simulink model "sampleModel1568"  (R2023a)
settings: Solver=VariableStepAuto  StartTime=0.0  StopTime=10.0  RelTol=1e-3
libraries: hdlsllib x6, simulink x2
settings Model: Creator=user1  LastModifiedBy=user1

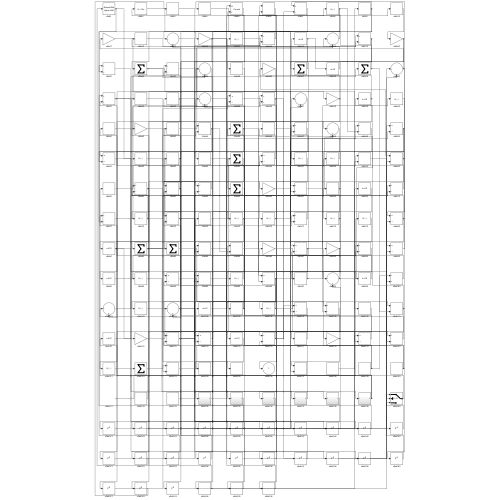
[thumbnail: Simulink's stored preview of the top-level diagram]
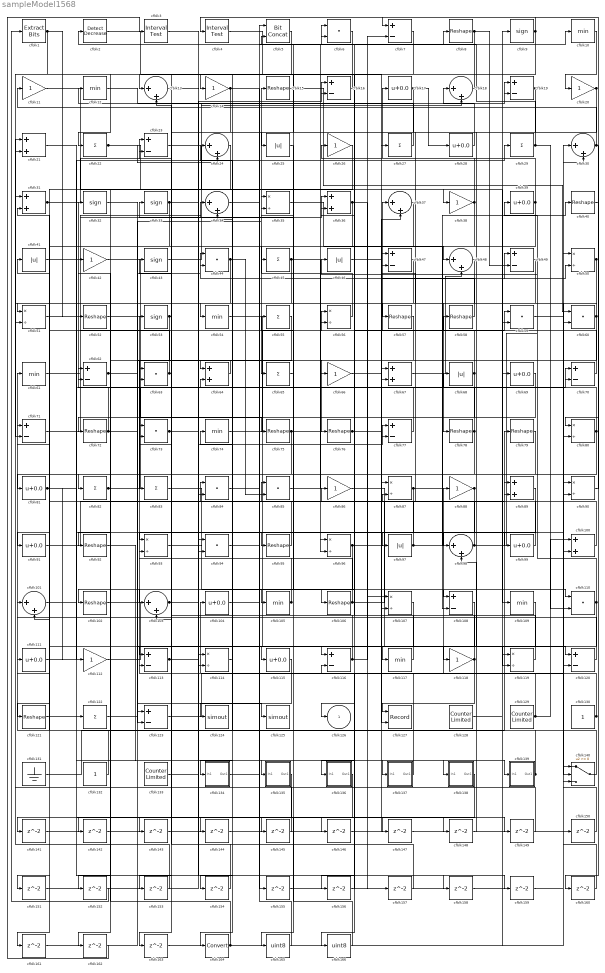
== system sampleModel1568 ==
  cfblk1 : simulink/Logic and Bit Operations/Extract Bits  bitsToExtract=Upper half  numBits=8  bitIdxRange=[0 7]  outScalingMode=Preserve fixed-point scaling
      settings: LibrarySourceBlock=|
      | hdlsllib/Logic and Bit
      | Operations/Extract Bits
  cfblk{10,12,54,61,74,105,109,117} (8 alike) : MinMax
  cfblk{21,31,36,64,67,89,100} (7 alike) : Sum
  cfblk{13,18,24,30,34,37,48,98,101,103} (10 alike) : Sum  Inputs=|++
  cfblk{8,15,40,52,57..58,72,75..76,78..79,92,95,102,106,121} (16 alike) : Reshape
  cfblk{17,28,39,69,81,91,99,104,111,115} (10 alike) : Bias  Bias=0.0  SaturateOnIntegerOverflow=off
  cfblk{35,50..51,56,80,87,90,93,96,107,114,119} (12 alike) : Product  Inputs=*/  RndMeth=Zero  SaturateOnIntegerOverflow=on
  cfblk{7,16,19,23,47,49,62,70..71,77,108,113,116,120,123} (15 alike) : Sum  Inputs=+-
  cfblk{11,14,20,26,38,42,66,86,88,112,118} (11 alike) : Gain
  cfblk{6,44,59..60,63,73,84..85,94,110} (10 alike) : DotProduct  OutDataTypeStr=Inherit: Inherit via internal rule
  cfblk{22,27,29,45,55,65,82..83,122} (9 alike) : Sum  Inputs=+
  cfblk124 : ToWorkspace  VariableName=simout  SaveFormat=Timeseries  SampleTime=-1
  cfblk125 : ToWorkspace  VariableName=simout  SaveFormat=Timeseries  SampleTime=-1
  cfblk127 : Record  FileSettingsInternal="{\"entries\":[{\"content\":{\"excelSettings\":{\"content\":{},\"type\":\"Streamout.ExcelSettings\"}},\"type\":\"Streamout.FileSettingStorage\",\"uuid\":\"\"}],\"packageUris\":[\"http:\\/\\/schema.mathworks.com\\/mf0\\/streamout_blocks\\/R2020a\"],\"version\":\"1.0\"}"  Layout=[1 1]  SignalsInternal="{\"entries\":[{\"content\":{},\"type\":\"RecordBlkView.InputSignals\",\"uuid\":\"\"}],\"packageUris\":[\"http:\\/\\/schema.mathworks.com\\/mf0\\/streamout_blocks\\/R2020a\"],\"version\":\"1.0\"}"  VisualizationBindings="{\"xyplotplugin\":{\"info\":[{\"series\":[{\"bindingParametersList\":[{\"parameter\":\"X-Axis\",\"signalID\":1822,\"signalName\":\"cfblk118\"},{\"parameter\":\"Y-Axis\",\"signalID\":1826,\"signalName\":\"cfblk49\"}],\"seriesID\":63146}],\"subplotID\":1}]}}"  CompatibilityTag=XY  st=-1
  cfblk128 : hdlsllib/Sources/Counter Limited  uplimit=7  tsamp=-1
  cfblk129 : hdlsllib/Sources/Counter Limited  uplimit=7  tsamp=-1
  cfblk130 : Constant  SampleTime=-1
  cfblk131 : Ground
  cfblk132 : Constant  SampleTime=-1
  cfblk133 : hdlsllib/Sources/Counter Limited  uplimit=7  tsamp=-1
  cfblk134 : Subsystem
      settings: LibrarySourceBlock=|
      | hdlsllib/Ports &
      | Subsystems/Subsystem
  cfblk135 : Subsystem
      settings: LibrarySourceBlock=|
      | hdlsllib/Ports &
      | Subsystems/Subsystem
  cfblk136 : Subsystem
      settings: LibrarySourceBlock=|
      | hdlsllib/Ports &
      | Subsystems/Subsystem
  cfblk137 : Subsystem
      settings: LibrarySourceBlock=|
      | hdlsllib/Ports &
      | Subsystems/Subsystem
  cfblk138 : Subsystem
      settings: LibrarySourceBlock=|
      | hdlsllib/Ports &
      | Subsystems/Subsystem
  cfblk139 : Subsystem
      settings: LibrarySourceBlock=|
      | hdlsllib/Ports &
      | Subsystems/Subsystem
  cfblk140 : Switch  SaturateOnIntegerOverflow=off  InputSameDT=off
  cfblk{141..163} (23 alike) : Delay  SampleTime=1
  cfblk164 : DataTypeConversion  SaturateOnIntegerOverflow=off  RndMeth=Floor
  cfblk165 : DataTypeConversion  OutDataTypeStr=uint8  SaturateOnIntegerOverflow=off  RndMeth=Floor
  cfblk166 : DataTypeConversion  OutDataTypeStr=uint8  SaturateOnIntegerOverflow=off  RndMeth=Floor
  cfblk2 : simulink/Logic and Bit Operations/Detect Decrease  vinit=0.0  OutDataTypeStr=boolean
      settings: LibrarySourceBlock=|
      | hdlsllib/Logic and Bit
      | Operations/Detect
      | Decrease
  cfblk{25,41,46,68,97} (5 alike) : Abs  SaturateOnIntegerOverflow=off
  cfblk3 : hdlsllib/Logic and Bit Operations/Interval Test  IntervalClosedRight=on  uplimit=0.5  IntervalClosedLeft=on  lowlimit=-0.5  OutDataTypeStr=boolean
  cfblk{9,32..33,43,53} (5 alike) : Signum
  cfblk4 : hdlsllib/Logic and Bit Operations/Interval Test  IntervalClosedRight=on  uplimit=0.5  IntervalClosedLeft=on  lowlimit=-0.5  OutDataTypeStr=boolean
  cfblk5 : hdlsllib/Logic and Bit Operations/Bit Concat  numInputs=2
  cfblk126 : Outport  VectorParamsAs1DForOutWhenUnconnected=off
  wires:
  cfblk54/1 -> cfblk120/1
  cfblk31/1 -> cfblk23/1, cfblk97/1
  cfblk77/1 -> cfblk33/1
  cfblk129/1 -> cfblk104/1, cfblk35/2, cfblk100/1
  cfblk16/1 -> cfblk13/1
  cfblk92/1 -> cfblk135/1(In1)
  cfblk121/1 -> cfblk122/1
  cfblk140/1 -> cfblk74/1
  cfblk132/1 -> cfblk61/1
  cfblk81/1 -> cfblk112/1, cfblk159/1
  cfblk74/1 -> cfblk59/1
  cfblk98/1 -> cfblk46/1, cfblk31/2
  cfblk131/1 -> cfblk79/1
  cfblk23/1 -> cfblk38/1
  cfblk42/1 -> cfblk64/1
  cfblk5/1 -> cfblk164/1
  cfblk102/1 -> cfblk116/1
  cfblk15/1 -> cfblk60/1
  cfblk118/1 -> cfblk127/1, cfblk43/1
  cfblk72/1 -> cfblk32/1, cfblk35/1
  cfblk73/1 -> cfblk145/1, cfblk146/1
  cfblk100/1 -> cfblk26/1
  cfblk33/1 -> cfblk114/1, cfblk81/1
  cfblk82/1 -> cfblk64/2, cfblk125/1, cfblk44/2
  cfblk56/1 -> cfblk15/1
  cfblk17/1 -> cfblk28/1, cfblk84/2
  cfblk26/1 -> cfblk82/1
  cfblk60/1 -> cfblk51/1, cfblk166/1
  cfblk43/1 -> cfblk19/1
  cfblk70/1 -> cfblk37/1
  cfblk123/1 -> cfblk30/1
  cfblk88/1 -> cfblk126/1, cfblk87/2
  cfblk115/1 -> cfblk124/1
  cfblk12/1 -> cfblk19/2
  cfblk90/1 -> cfblk4/1
  cfblk3/1 -> cfblk137/1(In1)
  cfblk29/1 -> cfblk2/1, cfblk110/2
  cfblk122/1 -> cfblk70/1
  cfblk57/1 -> cfblk76/1
  cfblk48/1 -> cfblk78/1
  cfblk68/1 -> cfblk134/1(In1), cfblk6/2
  cfblk41/1 -> cfblk36/1
  cfblk134/1(Out1) -> cfblk8/1
  cfblk91/1 -> cfblk89/1
  cfblk45/1 -> cfblk96/1, cfblk101/2
  cfblk119/1 -> cfblk86/1
  cfblk52/1 -> cfblk75/1
  cfblk78/1 -> cfblk96/2, cfblk34/2
  cfblk130/1 -> cfblk88/1, cfblk85/1
  cfblk25/1 -> cfblk95/1
  cfblk120/1 -> cfblk101/1
  cfblk35/1 -> cfblk48/1
  cfblk28/1 -> cfblk18/1
  cfblk67/1 -> cfblk48/2
  cfblk112/1 -> cfblk115/1
  cfblk103/1 -> cfblk114/2, cfblk16/1
  cfblk61/1 -> cfblk18/2
  cfblk37/1 -> cfblk123/2
  cfblk22/1 -> cfblk67/1, cfblk24/2
  cfblk128/1 -> cfblk9/1
  cfblk63/1 -> cfblk41/1, cfblk103/1
  cfblk137/1(Out1) -> cfblk53/1
  cfblk65/1 -> cfblk105/1
  cfblk85/1 -> cfblk10/1
  cfblk94/1 -> cfblk138/1(In1)
  cfblk110/1 -> cfblk39/1, cfblk154/1
  cfblk114/1 -> cfblk24/1
  cfblk20/1 -> cfblk118/1, cfblk103/2
  cfblk38/1 -> cfblk17/1, cfblk72/1
  cfblk133/1 -> cfblk77/1
  cfblk18/1 -> cfblk14/1
  cfblk55/1 -> cfblk83/1
  cfblk62/1 -> cfblk119/2, cfblk142/1
  cfblk104/1 -> cfblk56/1
  cfblk105/1 -> cfblk102/1, cfblk93/2
  cfblk76/1 -> cfblk50/2, cfblk36/2
  cfblk58/1 -> cfblk44/1
  cfblk80/1 -> cfblk62/1, cfblk141/1
  cfblk96/1 -> cfblk99/1, cfblk143/1, cfblk144/1
  cfblk19/1 -> cfblk57/1, cfblk107/2
  cfblk49/1 -> cfblk127/2
  cfblk71/1 -> cfblk58/1
  cfblk44/1 -> cfblk51/2, cfblk85/2
  cfblk1/1 -> cfblk21/2, cfblk52/1
  cfblk117/1 -> cfblk34/1
  cfblk14/1 -> cfblk117/1, cfblk16/2, cfblk113/1
  cfblk106/1 -> cfblk89/2, cfblk73/2
  cfblk93/1 -> cfblk108/1
  cfblk46/1 -> cfblk67/2
  cfblk9/1 -> cfblk54/1, cfblk7/1, cfblk71/2
  cfblk11/1 -> cfblk109/1
  cfblk86/1 -> cfblk140/2
  cfblk79/1 -> cfblk106/1
  cfblk4/1 -> cfblk27/1
  cfblk95/1 -> cfblk84/1
  cfblk27/1 -> cfblk12/1
  cfblk36/1 -> cfblk65/1, cfblk157/1
  cfblk6/1 -> cfblk22/1
  cfblk113/1 -> cfblk56/2, cfblk68/1, cfblk158/1
  cfblk116/1 -> cfblk45/1, cfblk7/2, cfblk107/1
  cfblk111/1 -> cfblk70/2
  cfblk7/1 -> cfblk25/1
  cfblk75/1 -> cfblk121/1, cfblk100/2
  cfblk59/1 -> cfblk90/1
  cfblk64/1 -> cfblk63/1
  cfblk53/1 -> cfblk13/2, cfblk162/1
  cfblk32/1 -> cfblk66/1
  cfblk50/1 -> cfblk98/1, cfblk120/2
  cfblk66/1 -> cfblk77/2
  cfblk2/1 -> cfblk87/1
  cfblk39/1 -> cfblk108/2, cfblk6/1
  cfblk139/1(Out1) -> cfblk111/1, cfblk71/1, cfblk62/2
  cfblk69/1 -> cfblk92/1
  cfblk10/1 -> cfblk20/1
  cfblk30/1 -> cfblk80/1, cfblk11/1
  cfblk21/1 -> cfblk139/1(In1)
  cfblk83/1 -> cfblk110/1
  cfblk97/1 -> cfblk55/1, cfblk40/1
  cfblk8/1 -> cfblk93/1, cfblk136/1(In1), cfblk49/2
  cfblk24/1 -> cfblk91/1
  cfblk47/1 -> cfblk73/1
  cfblk101/1 -> cfblk29/1
  cfblk99/1 -> cfblk47/1
  cfblk87/1 -> cfblk94/2, cfblk49/1
  cfblk141/1 -> cfblk30/2
  cfblk142/1 -> cfblk37/2
  cfblk143/1 -> cfblk59/2
  cfblk144/1 -> cfblk90/2
  cfblk145/1 -> cfblk21/1
  cfblk146/1 -> cfblk47/2
  cfblk34/1 -> cfblk147/1
  cfblk147/1 -> cfblk119/1
  cfblk13/1 -> cfblk148/1
  cfblk148/1 -> cfblk98/2
  cfblk51/1 -> cfblk149/1
  cfblk149/1 -> cfblk23/2
  cfblk150/1 -> cfblk50/1
  cfblk138/1(Out1) -> cfblk151/1
  cfblk151/1 -> cfblk94/1
  cfblk108/1 -> cfblk152/1
  cfblk152/1 -> cfblk1/1
  cfblk89/1 -> cfblk153/1
  cfblk153/1 -> cfblk31/1
  cfblk154/1 -> cfblk63/2
  cfblk84/1 -> cfblk155/1
  cfblk155/1 -> cfblk60/2
  cfblk107/1 -> cfblk156/1
  cfblk156/1 -> cfblk116/2
  cfblk157/1 -> cfblk113/2
  cfblk158/1 -> cfblk80/2
  cfblk159/1 -> cfblk140/3
  cfblk40/1 -> cfblk160/1
  cfblk160/1 -> cfblk140/1
  cfblk109/1 -> cfblk161/1
  cfblk161/1 -> cfblk123/1
  cfblk162/1 -> cfblk3/1
  cfblk135/1(Out1) -> cfblk163/1
  cfblk163/1 -> cfblk69/1
  cfblk164/1 -> cfblk150/1, cfblk42/1
  cfblk136/1(Out1) -> cfblk165/1
  cfblk165/1 -> cfblk5/1
  cfblk166/1 -> cfblk5/2

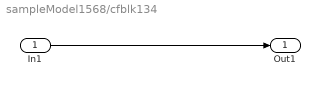
== system sampleModel1568/cfblk134 ==
  In1 : Inport
  Out1 : Outport
  wires:
  In1/1 -> Out1/1

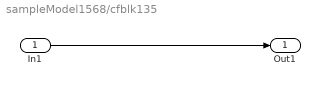
== system sampleModel1568/cfblk135 ==
  In1 : Inport
  Out1 : Outport
  wires:
  In1/1 -> Out1/1

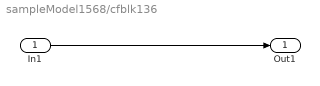
== system sampleModel1568/cfblk136 ==
  In1 : Inport
  Out1 : Outport
  wires:
  In1/1 -> Out1/1

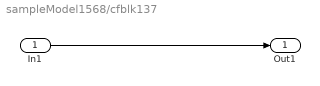
== system sampleModel1568/cfblk137 ==
  In1 : Inport
  Out1 : Outport
  wires:
  In1/1 -> Out1/1

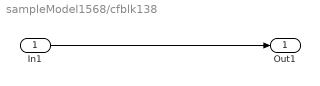
== system sampleModel1568/cfblk138 ==
  In1 : Inport
  Out1 : Outport
  wires:
  In1/1 -> Out1/1

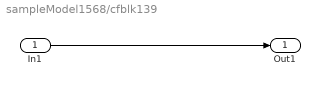
== system sampleModel1568/cfblk139 ==
  In1 : Inport
  Out1 : Outport
  wires:
  In1/1 -> Out1/1
